simulink model "untitled1"  (R2018b)
settings: Solver=FixedStepAuto  StartTime=0.0  StopTime=1  FixedStep=1/400  RelTol=1e-3
libraries: libslotcar x3, simulink x1
settings Model: Creator=Lenovo  LastModifiedBy=Lenovo

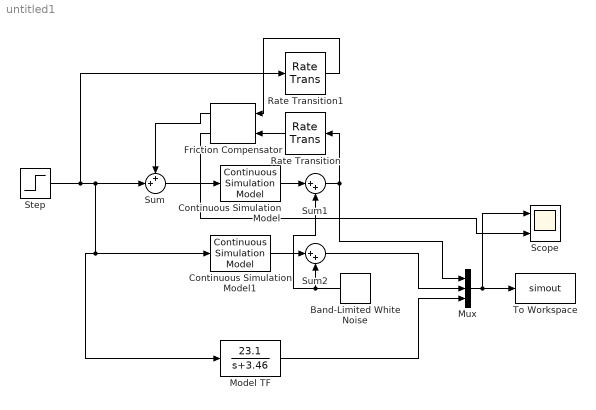
== system untitled1 ==
  Band-Limited White Noise : simulink/Sources/Band-Limited White Noise  Cov=[0.0001]  Ts=1/400  seed=[23341]
  Continuous Simulation Model : libslotcar/Continuous Simulation Model  tsparam=-1  mparam=0.173  dparam=0.018  nparam=9/28  uparam=12.25-0.7  rparam=5  kparam=0.005  ksparam=0.7183  kdparam=0.3415
  Continuous Simulation Model1 : libslotcar/Continuous Simulation Model  tsparam=-1  mparam=0.173  dparam=0.018  nparam=9/28  uparam=12.25-0.7  rparam=5  kparam=0.005  ksparam=0.7183  kdparam=0.3415
  Friction Compensator : libslotcar/Friction Compensator  coul=0.7183  visc=0.3415  A=-3.4  B=23  Q=1  R=1  Gain=1/3.9963
  Model TF : TransferFcn  Numerator=23.1  Denominator=[1 3.46]  ContinuousStateAttributes='velocity'
  Mux : Mux  Inputs=3
  Rate Transition : RateTransition  OutPortSampleTimeOpt=Inherit
  Rate Transition1 : RateTransition  OutPortSampleTimeOpt=Inherit
  Scope : Scope  NumInputPorts=2
  Step : Step  Time=0  SampleTime=0
  Sum : Sum  Inputs=++|
  Sum1 : Sum  Inputs=|++
  Sum2 : Sum  Inputs=|++
  To Workspace : ToWorkspace  VariableName=simout  SaveFormat=Timeseries  SampleTime=-1
  wires:
  Step/1 -> Rate Transition1/1, Model TF/1, Continuous Simulation Model1/1, Sum/2
  Sum/1 -> Continuous Simulation Model/1
  Friction Compensator/1 -> Sum/1
  Mux/1 -> Scope/1, To Workspace/1
  Continuous Simulation Model/1 -> Sum1/1
  Sum1/1 -> Mux/1, Rate Transition/1
  Band-Limited White Noise/1 -> Sum1/2, Sum2/2
  Continuous Simulation Model1/1 -> Sum2/1
  Model TF/1 -> Mux/3
  Sum2/1 -> Mux/2
  Rate Transition/1 -> Friction Compensator/2
  Rate Transition1/1 -> Friction Compensator/1
  Friction Compensator/2 -> Scope/2
